simulink model "SVM_sim"  (R2018b)
settings: Solver=VariableStepAuto  StartTime=0.0  StopTime=Inf  FixedStep=T/4  RelTol=1e-3
PostLoadFcn:
  | , if any(exist('dsrtsu_mdlpostloadfcn', 'file') ~= 0), dsrtsu_mdlpostloadfcn('Execute', bdroot); end,
values from neighbouring files (symbols this model uses):
  fixed_io_gain = 175    [parameters.m]
  fixed_vclamp_gain = 1000    [parameters.m]
  fixed_vi_gain = 5800    [parameters.m]
  ioa_gain = 1    [parameters.m]
  ioa_offset = -39.67    [parameters.m]
  iob_gain = 1    [parameters.m]
  iob_offset = -40.05    [parameters.m]
  ioc_gain = 1    [parameters.m]
  ioc_offset = -39.51    [parameters.m]
  N = 500    [parameters.m]
  phi = 0    [parameters.m]
  threshold = 100    [parameters.m]
  vclamp_gain = 1    [parameters.m]
  vclamp_offset = -0.9    [parameters.m]
  via_gain = 1    [parameters.m]
  via_offset = -836.4    [parameters.m]
  vib_gain = 1    [parameters.m]
  vib_offset = -854.9    [parameters.m]
  vic_gain = 1    [parameters.m]
  vic_offset = -852.3    [parameters.m]
libraries: xbsIndex_r4 x465, rtiproclib x10, rti1202lib_adc_class1 x8, simulink x4, powerlib_meascontrol x1, rtifpgainterfacelib x1
(part 2 of 9)

== system SVM_sim/RTI Data ==
  RTI Data Store : Subsystem  Tag="struct('private',struct('version',struct('dsVer',uint32(2),'dsVerCreation',uint32(2),'RTI',struct('ver','7.13','type','RTI1202')),'access',struct('type','Model','isPerm',1,'created',['06-Mar-2025 17:54:56'],'modified',['07-Mar-2025 16:09:59'],'location','')),'public',struct('main',struct('data',[]),'sub',struct('name',{{'SVM_sim'}},'data',{{struct('TH',struct('thTaskInfo',struct('taskType',{'TIMER','HWINT','TMRINT','SWINT','GLINT'},'tasksNumOf',{1,2,0,0,0},'srcIds',{{'TIMERA'},{'FPGACL1FPGA_INTP0Ch0','FPGACL1FPGA_INTP0Ch1'},{},{},{}},'taskNames',{{['Timer Task 1']},{'PROC_INT_BL1','PROC_INT_BL2'},{},{},{}})),'th_tc',struct('dataType',{'TASK','TASK','TASK'},'taskGroupId',{'','',''},'taskGroupList',{{},{},{}},'taskSchedulingPolicy',{'FCFS','FCFS','FCFS'},'taskType',{'TIMER','HWINT','HWINT'},'blkh',{-1,['SVM_sim/PROC_INT_BL1/Common Hardware' char(10) 'Interrupt Interface'],['SVM_sim/PROC_INT_BL2/Common Hardware' char(10) 'Interrupt Interface']},'srcId',{'TIMERA','FPGACL1FPGA_INTP0Ch0','FPGACL1FPGA_INTP0Ch1'},'srcSgnName',{['Timer A interrupt'],['FPGA Type CL1 FPGA_INT Port 0 Channel 0'],['FPGA Type CL1 FPGA_INT Port 0 Channel 1']},'srcCpuName',{'','',''},'taskName',{['Timer Task 1  [0.00025] s'],'PROC_INT_BL1','PROC_INT_BL2'},'taskNameDisplayExt',{'','',''},'smplTime',{0.00025,0,0},'smplTimeOffs',{0,0,0},'hasFixedPriority',{0,0,0},'priority',{1,2,3},'hasFixedOvc',{0,0,0},'ovcType',{1,1,1},'ovcMax',{1,1,1}),'tc_th',struct('dataType',{'TASK','TASK','TASK'},'taskGroupId',{'','',''},'taskGroupList',{{},{},{}},'taskSchedulingPolicy',{'FCFS','FCFS','FCFS'},'taskType',{'TIMER','HWINT','HWINT'},'blkh',{-1,['SVM_sim/PROC_INT_BL1/Common Hardware' char(10) 'Interrupt Interface'],['SVM_sim/PROC_INT_BL2/Common Hardware' char(10) 'Interrupt Interface']},'srcId',{'TIMERA','FPGACL1FPGA_INTP0Ch0','FPGACL1FPGA_INTP0Ch1'},'srcSgnName',{['Timer A interrupt'],['FPGA Type CL1 FPGA_INT Port 0 Channel 0'],['FPGA Type CL1 FPGA_INT Port 0 Channel 1']},'srcCpuName',{'','',''},'taskName',{['Timer Task 1  [0.00025] s'],'PROC_INT_BL1','PROC_INT_BL2'},'taskNameDisplayExt',{'','',''},'smplTime',{0.00025,0,0},'smplTimeOffs',{0,0,0},'hasFixedPriority',{0,0,0},'priority',{1,2,3},'hasFixedOvc',{0,0,0},'ovcType',{1,1,1},'ovcMax',{1,1,1}))}})))"  mask(RTI_DATA_STORE){}
      mask help:
      | RTI Data Store Block. This block is used by RTI to store internal model dependent data. Deleting this block will result in data loss.
      |
      | NEVER DELETE, COPY, OR MODIFY THIS BLOCK!
      mask Help:
      | RTI Data Store Block. This block is used by RTI to store internal model dependent data. Deleting this block will result in data loss.
      | 
      | NEVER DELETE, COPY, OR MODIFY THIS BLOCK!
      mask Display: text(0.5, 0.5, ' ', 'HorizontalAlignment', 'center');

== system SVM_sim/Subsystem ==
  a_hat : Inport
  b_hat : Inport  Port=2
  phi : Inport  Port=3
  q : Inport  Port=4
  Kv : Inport  Port=5
  Ki : Inport  Port=6
  function : TriggerPort  TriggerType=function-call  VariantControl=Variant
  MATLAB Function2 : MATLAB Function  TreatAsAtomicUnit=on
  MATLAB Function3 : MATLAB Function  TreatAsAtomicUnit=on
  d1 : Outport
  d2 : Outport  Port=2
  d3 : Outport  Port=3
  d4 : Outport  Port=4
  set : Outport  Port=5
  wires:
  MATLAB Function2/2(d2) -> d2/1
  b_hat/1 -> MATLAB Function2/2(b_hat)
  MATLAB Function2/4(d4) -> d4/1
  phi/1 -> MATLAB Function2/3(phi)
  MATLAB Function2/3(d3) -> d3/1
  q/1 -> MATLAB Function2/4(q)
  a_hat/1 -> MATLAB Function2/1(a_hat)
  MATLAB Function2/1(d1) -> d1/1
  MATLAB Function3/1(set) -> set/1
  Ki/1 -> MATLAB Function3/2(Ki)
  Kv/1 -> MATLAB Function3/1(Kv)

== system SVM_sim/Subsystem1 ==
  function : TriggerPort  TriggerType=function-call  VariantControl=Variant
